simulink model "sf_ifelse"  (R2015b)
settings: Solver=FixedStepDiscrete  SolverMode=SingleTasking  StartTime=0.0  StopTime=1/5  RelTol=1e-3
settings Model: Creator=at-mt  LastModifiedBy=amatsumo
settings DataIOCC: SaveFormat=Array  SignalLoggingSaveFormat=ModelDataLogs  SaveOutput=off  SignalLogging=off  SaveTime=off
settings OptimizationCC: BlockReduction=off  ConditionallyExecuteInputs=off  DefaultParameterBehavior=Inlined  ExpressionDepthLimit=2147483647
settings DebuggingCC: AlgebraicLoopMsg=error  UnderspecifiedInitializationDetection=Classic  MergeDetectMultiDrivingBlocksExec=none  SolverPrmCheckMsg=warning  SingleTaskRateTransMsg=error  FcnCallInpInsideContextMsg=UseLocalSettings  StateNameClashWarn=warning
settings HardwareCC: ProdBitPerPointer=32  ProdLargestAtomicFloat=None  ProdIntDivRoundTo=Undefined  ProdEndianess=Unspecified  ProdWordSize=32  ProdHWDeviceType=ASIC/FPGA->ASIC/FPGA  ProdEqTarget=off
settings GRTTargetCC: GeneratePreprocessorConditionals=Disable all  CombineOutputUpdateFcns=off  GRTInterface=on
settings ConfigComp: CovMetricSettings=dcmw  CovSFcnEnable=off

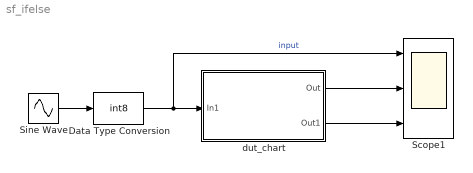
== system sf_ifelse ==
  Data Type Conversion : DataTypeConversion  OutDataTypeStr=int8
  Scope1 : Scope  NumInputPorts=3
  Sine Wave : Sin  Amplitude=127  Frequency=2*pi*10  SampleTime=1/100
  dut_chart : Subsystem
  wires:
  Sine Wave/1 -> Data Type Conversion/1
  Data Type Conversion/1 -> Scope1/1, dut_chart/1(In1)  "input"
  dut_chart/1(Out) -> Scope1/2
  dut_chart/2(Out1) -> Scope1/3

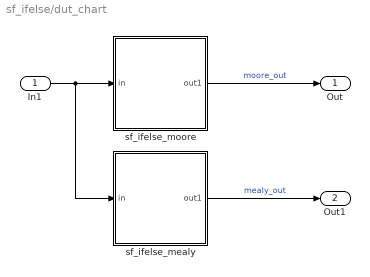
== system sf_ifelse/dut_chart ==
  In1 : Inport
  sf_ifelse_mealy : Stateflow chart  TreatAsAtomicUnit=on
  sf_ifelse_moore : Stateflow chart  TreatAsAtomicUnit=on
  Out : Outport
  Out1 : Outport  Port=2
  wires:
  In1/1 -> sf_ifelse_moore/1(in), sf_ifelse_mealy/1(in)
  sf_ifelse_moore/1(out1) -> Out/1  "moore_out"
  sf_ifelse_mealy/1(out1) -> Out1/1  "mealy_out"

== stateflow chart sf_ifelse/dut_chart/sf_ifelse_mealy ==
  settings: updateMethod=DISCRETE  stateMachineType=MEALY_MACHINE  executeAtInitialization=1
  state Init/
  state On1/
  Init -> Init [order 2] : {out1 = out1;}
  (default) -> Init
  Init -> On1 [order 1] : [in < 0]
      | {out1 = 1;}
  On1 -> Init [order 1] : [in >= 0]
      | {out1 = 2;}
  On1 -> On1 [order 2] : {out1 = 1;}
  data: in input int8 size=1; out1 output int8

== stateflow chart sf_ifelse/dut_chart/sf_ifelse_moore ==
  settings: updateMethod=DISCRETE  stateMachineType=MOORE_MACHINE  executeAtInitialization=1
  state Init/
    out1 = 2;
  state On1/
    out1 = 1;
  Init -> Init [order 2]
  (default) -> Init
  Init -> On1 [order 1] : [in < 0]
  On1 -> Init [order 1] : [in >= 0]
  On1 -> On1 [order 2]
  data: in input int8 size=1; out1 output int8
